simulink model "tqdtqr_rebuild_V3"  (R2021b)
settings: Solver=VariableStepAuto  StartTime=0.0  StopTime=10.0  RelTol=1e-3
undefined symbols (not defined in the file): ATQD_AfterTqMinGain_X_Deg, ATQD_APSCreepBaseTqD_X_kph, ATQD_APSCreepBaseTqD_Y_Deg, ATQD_APSCreepBaseTqR_X_kph, ATQD_APSCreepBaseTqR_Y_Deg, ATQD_APSCreepIterm_X_kph, ATQD_APSCreepIterm_Y_kph, ATQD_APSCreepPterm_X_kph, ATQD_APSCreepPterm_Y_kph, ATQD_APSDecReq_X_kph, ATQD_APSDecReq_Y_mps2, ATQD_APSDecReqCMD_X_kph, ATQD_APSDecReqTs_X_pct, ATQD_APSDecTimeGain_X_Deg, ATQD_APSDecTimeGain_Y_s, ATQD_APSReqLowSpd_X_Deg, ATQD_AutoHoldReleaseBPS_X_Deg, ATQD_AWDLoadTrqnsGain_X_kg, ATQD_AWDLoadTrqnsGain_Y_pct, ATQD_BOSEnBPSPosn_X_kph, ATQD_BOSMap_X_rpm, ATQD_BOSMap_Y_pct, ATQD_CreepBaseTqD_X_kph, ATQD_CreepBaseTqD_Y_Deg, ATQD_CreepBaseTqR_X_kph, ATQD_CreepBaseTqR_Y_Deg, ATQD_CreepBPSDisPosn_X_Deg, ATQD_CreepBPSDisPosnR_X_Deg, ATQD_CreepBPSEnPosn_X_Deg, ATQD_CreepBPSEnPosnR_X_Deg, ATQD_CreepDeltaTq_X_kph, ATQD_CreepIterm_X_kph, ATQD_CreepIterm_Y_kph, ATQD_CreepItermMaxLimit_X_pct, ATQD_CreepPreloadTime_X_kph, ATQD_CreepPreloadTq_X_kph, ATQD_CreepPreloadTq_Y_s, ATQD_CreepProtTq_X_Deg, ATQD_CreepPterm_X_kph, ATQD_CreepPterm_Y_kph, ATQD_CreepRrTqSpRat_X_rpm, ATQD_CreepRrTqSpRat_Y_Nm, ATQD_CreepTargetSpdD_X_pct, ATQD_CreepTargetSpdR_X_pct, ATQD_CreepUpLimitTq_X_rpm, ATQD_DecIneOPDHoldEnDelay_X_Deg, ATQD_DecIneOPDHoldEnDelay_Y_bar, ATQD_ECOTqMapD_X_rpm, ATQD_ECOTqMapD_Y_pct, ATQD_EMTqMapD_X_rpm, ATQD_EMTqMapD_Y_pct, ATQD_EOPDTqMapDCon_X_rpm, ATQD_EOPDTqMapDCon_Y_Deg, ATQD_EstInitVehWeight_X_c, ATQD_FAfterTqCMDGain_X_rpm, ATQD_FAfterTqCMDGain_Y_pct, ATQD_ForceLowSpd_X_Deg, ATQD_ForcePLimitSpd_X_Deg, ATQD_FrLossMAPLowV_X_rpm, ATQD_FrLossMAPLowV_Y_Nm ... (+949)
libraries: simulink x235, hcu_lib x208, tqr x63, tqd x6
(part 15 of 37)

== system tqdtqr_rebuild_V3/Input_Convert/Main function/AvaliableTqLimit function/TorqueCapacityCalcalation ==
  VTQD_FrShaftSpd_rpm : Inport
  VTQD_RrShaftSpd_rpm : Inport  Port=2
  VINP_HVBPwrAvailDchrg_kw : Inport  Port=3
  VINP_HVBPwrAvailChrg_kw : Inport  Port=4
  KTQD_FrBatapCont_factor : Inport  Port=5
  KTQD_RrBatapCont_factor : Inport  Port=6
  VTQD_FrEDUSpRat_cmd : Inport  Port=7
  VTQD_RrEDUSpRat_rat : Inport  Port=8
  VINP_FrMotorAvailTq_Nm : Inport  Port=9
  VINP_RrMotorAvailTq_Nm : Inport  Port=10
  VINP_FrRegenAvailTq_Nm : Inport  Port=11
  VINP_RrRegenAvailTq_Nm : Inport  Port=12
  VTQD_GearActualPosn_enum : Inport  Port=13
  VINP_VehicleType_enum : Inport  Port=14
  VTQD_CoordWhlTqDemFr_Nm : Inport  Port=15
  VTQD_CoordWhlTqDemRr_Nm : Inport  Port=16
  VINP_FrMCUDCBusVolt_V : Inport  Port=17
  VINP_RrMCUDCBusVolt_V : Inport  Port=18
  VPMM_DrivetrainSelect_enum : Inport  Port=19
  VINP_FrMCUTemp_C : Inport  Port=20
  VINP_FrTMTemp_C : Inport  Port=21
  VINP_RrMCUTemp_C : Inport  Port=22
  VINP_RrTMTemp_C : Inport  Port=23
  VTQD_IVIRockModeEn_flg : Inport  Port=24
  VTQD_ActAPSPosn_pct : Inport  Port=25
  task_time_s : Inport  Port=26
  CapacityDistribution : Subsystem
  Constant1 : Constant  Value=KTQD_RockInitMotTqInc_Nm
  Constant10 : Constant  Value=KTQD_RrUppTheldTrq_Nm
  Constant11 : Constant  Value=KTQD_RrUppTheldTrq_Nm
  Constant12 : Constant  Value=KTQD_RockInitTqMotDec_Nm
  Constant13 : Constant  Value=KTQD_RockAvalMotTqReset_pct
  Constant14 : Constant  Value=KTQD_RockAvalMotTqReset_pct
  Constant2 : Constant  Value=KTQD_FrRockAvalMotTqInc_Nm
  Constant3 : Constant  Value=KTQD_FrRockAvalMotBaseTq_Nm
  Constant4 : Constant  Value=KTQD_FrUppTheldTrq_Nm
  Constant5 : Constant  Value=KTQD_FrUppTheldTrq_Nm
  Constant6 : Constant  Value=KTQD_RockInitTqMotDec_Nm
  Constant7 : Constant  Value=KTQD_RockInitMotTqInc_Nm
  Constant8 : Constant  Value=KTQD_RrRockAvalMotTqInc_Nm
  Constant9 : Constant  Value=KTQD_RrRockAvalMotBaseTq_Nm
  Generation : tqd/TQD/TorqueDemand/TorqueModule/AvaliableTqLimit/TorqueCapacityCalcalation/Generation  SystemSampleTime=-1  VariantActivationTime=update diagram  Latency=0  AutoFrameSizeCalculation=off
  KTQD_FrMotorTempHigh_C KTQD_FrMotorTempLow_C : Relay  OnSwitchValue=KTQD_FrMotorTempHigh_C  OffSwitchValue=KTQD_FrMotorTempLow_C  OutDataTypeStr=boolean
  KTQD_RrMotorTempHigh_C KTQD_RrMotorTempLow_C : Relay  OnSwitchValue=KTQD_RrMotorTempHigh_C  OffSwitchValue=KTQD_RrMotorTempLow_C  OutDataTypeStr=boolean
  "MOTOR Loss MAP " : Subsystem
  MTQD_FrGenActReduce_Z_Nm : Lookup_n-D  BreakpointsForDimension1=ATQD_FrMotActReduce_Y_C  BreakpointsForDimension2=ATQD_FrMotActReduce_X_rpm  Table=MTQD_FrGenActReduce_Z_Nm  InternalRulePriority=Speed  RndMeth=Simplest  InputSameDT=on
      settings: InputPortMap=u0,u1
  MTQD_FrMotActReduce_Z_Nm : Lookup_n-D  BreakpointsForDimension1=ATQD_FrMotActReduce_Y_C  BreakpointsForDimension2=ATQD_FrMotActReduce_X_rpm  Table=MTQD_FrMotActReduce_Z_Nm  InternalRulePriority=Speed  RndMeth=Simplest  InputSameDT=on
      settings: InputPortMap=u0,u1
  MTQD_RrGenActReduce_Z_Nm : Lookup_n-D  BreakpointsForDimension1=ATQD_FrMotActReduce_Y_C  BreakpointsForDimension2=ATQD_FrMotActReduce_X_rpm  Table=MTQD_RrGenActReduce_Z_Nm  InternalRulePriority=Speed  RndMeth=Simplest  InputSameDT=on
      settings: InputPortMap=u0,u1
  MTQD_RrMotActReduce_Z_Nm : Lookup_n-D  BreakpointsForDimension1=ATQD_FrMotActReduce_Y_C  BreakpointsForDimension2=ATQD_FrMotActReduce_X_rpm  Table=MTQD_RrMotActReduce_Z_Nm  InternalRulePriority=Speed  RndMeth=Simplest  InputSameDT=on
      settings: InputPortMap=u0,u1
  Max{,1..7} (8 alike) : MinMax  Function=max  Inputs=2
  Motoring : tqd/TQD/TorqueDemand/TorqueModule/AvaliableTqLimit/TorqueCapacityCalcalation/Motoring  SystemSampleTime=-1  VariantActivationTime=update diagram  Latency=0  AutoFrameSizeCalculation=off
  OR : Logic  Operator=OR  AllPortsSameDT=off  OutDataTypeStr=boolean
  OR1 : Logic  Operator=OR  AllPortsSameDT=off  OutDataTypeStr=boolean
  RateLimit : hcu_lib/Basic_Blocks/RateLimit
  RateLimit1 : hcu_lib/Basic_Blocks/RateLimit
  Relational Operator : RelationalOperator  Operator=<=  OutDataTypeStr=boolean  RndMeth=Simplest
  Relational Operator1 : RelationalOperator  Operator=<=  OutDataTypeStr=boolean  RndMeth=Simplest
  Switch{,1..3} (4 alike) : Switch  Criteria=u2 ~= 0
      settings: AttributesFormatString=%<Criteria>
  TMAvailablePwr_Calculation : Subsystem
  VTQD_WhlTqCapMotFr_Nm : Outport
  VTQD_WhlTqCapMotRr_Nm : Outport  Port=2
  VTQD_WhlTqCapGenFr_Nm : Outport  Port=3
  VTQD_WhlTqCapGenRr_Nm : Outport  Port=4
  VTQD_MotorLossTotal_kw : Outport  Port=5
  wires:
  [VTQD_TMPwrAvailDchrg_kW] -> CapacityDistribution/3(VTQD_TMPwrAvailDchrg_kW)
  TMAvailablePwr_Calculation/1(VTQD_TMPwrAvailDchrg_kW) -> [VTQD_TMPwrAvailDchrg_kW]
  [VINP_HVBPwrAvailDchrg_kw] -> TMAvailablePwr_Calculation/1(VINP_HVBPwrAvailDchrg_kw)
  Motoring/2 -> VTQD_WhlTqCapMotRr_Nm/1
  [VTQD_RrEDUSpRat_rat] -> CapacityDistribution/2(VTQD_RrEDUSpRat_rat)
  [VTQD_FrEDUSpRat_rat] -> CapacityDistribution/1(VTQD_FrEDUSpRat_cmd)
  CapacityDistribution/4(VTQD_RrHVBPwrAvailChrg_kw) -> [VTQD_RrHVBPwrAvailChrg_kw]
  CapacityDistribution/3(VTQD_FrHVBPwrAvailChrg_kw) -> [VTQD_FrHVBPwrAvailChrg_kw]
  CapacityDistribution/2(VTQD_RrHVBPwrAvailDchrg_kw) -> [VTQD_RrHVBPwrAvailDchrg_kw]
  CapacityDistribution/1(VTQD_FrHVBPwrAvailDchrg_kw) -> [VTQD_FrHVBPwrAvailDchrg_kw]
  [VINP_HVBPwrAvailChrg_kw] -> CapacityDistribution/4(VINP_HVBPwrAvailChrg_kw)
  Generation/1 -> VTQD_WhlTqCapGenFr_Nm/1
  VTQD_RrEDUSpRat_rat/1 -> [VTQD_RrEDUSpRat_rat]
  VTQD_FrEDUSpRat_cmd/1 -> [VTQD_FrEDUSpRat_rat]
  KTQD_RrBatapCont_factor/1 -> [KTQD_RrBatapCont_factor]
  VTQD_RrShaftSpd_rpm/1 -> [VTQD_RrShaftSpd_rpm]
  VTQD_FrShaftSpd_rpm/1 -> [VTQD_FrShaftSpd_rpm]
  VINP_HVBPwrAvailChrg_kw/1 -> [VINP_HVBPwrAvailChrg_kw]
  VINP_HVBPwrAvailDchrg_kw/1 -> [VINP_HVBPwrAvailDchrg_kw]
  KTQD_FrBatapCont_factor/1 -> [KTQD_FrBatapCont_factor]
  Motoring/1 -> VTQD_WhlTqCapMotFr_Nm/1
  VINP_RrRegenAvailTq_Nm/1 -> [VINP_RrRegenAvailTq_Nm]
  VINP_FrRegenAvailTq_Nm/1 -> [VINP_FrRegenAvailTq_Nm]
  VINP_FrMotorAvailTq_Nm/1 -> [VINP_FrMotorAvailTq_Nm]
  VINP_RrMotorAvailTq_Nm/1 -> [VINP_RrMotorAvailTq_Nm]
  VTQD_GearActualPosn_enum/1 -> [VTQD_GearActualPosn_enum]
  VINP_VehicleType_enum/1 -> [VINP_VehicleType_enum]
  [VTQD_FrShaftSpd_rpm] -> "MOTOR Loss MAP "/1(VTQD_FrShaftSpd_rpm)
  [VTQD_RrShaftSpd_rpm] -> "MOTOR Loss MAP "/2(VTQD_RrShaftSpd_rpm)
  [VTQD_CoordWhlTqDemFr_Nm] -> "MOTOR Loss MAP "/3(VTQD_CoordWhlTqDemFr_Nm)
  [VTQD_CoordWhlTqDemRr_Nm] -> "MOTOR Loss MAP "/4(VTQD_CoordWhlTqDemRr_Nm)
  [VINP_FrMCUDCBusVolt_V] -> "MOTOR Loss MAP "/5(VINP_FrMCUDCBusVolt_V)
  [VINP_RrMCUDCBusVolt_V] -> "MOTOR Loss MAP "/6(VINP_RrMCUDCBusVolt_V)
  [VPMM_DrivetrainSelect_enum] -> "MOTOR Loss MAP "/7(VPMM_DrivetrainSelect_enum)
  VTQD_CoordWhlTqDemRr_Nm/1 -> [VTQD_CoordWhlTqDemRr_Nm]
  VTQD_CoordWhlTqDemFr_Nm/1 -> [VTQD_CoordWhlTqDemFr_Nm]
  VINP_FrMCUDCBusVolt_V/1 -> [VINP_FrMCUDCBusVolt_V]
  VINP_RrMCUDCBusVolt_V/1 -> [VINP_RrMCUDCBusVolt_V]
  VPMM_DrivetrainSelect_enum/1 -> [VPMM_DrivetrainSelect_enum]
  "MOTOR Loss MAP "/1(VTQD_MotorLossTotal_kW) -> VTQD_MotorLossTotal_kw/1, [VTQD_MotorLossTotal_kw]
  [VTQD_MotorLossTotal_kw] -> CapacityDistribution/5(VTQD_MotorLossTotal_kw)
  VINP_FrMCUTemp_C/1 -> [VINP_FrMCUTemp_C]
  VINP_FrTMTemp_C/1 -> [VINP_FrTMTemp_C]
  VINP_RrMCUTemp_C/1 -> [VINP_RrMCUTemp_C]
  VINP_RrTMTemp_C/1 -> [VINP_RrTMTemp_C]
  [VTQD_CoordWhlTqDemFr_Nm] -> Max6/2
  Constant3/1 -> Max6/1
  Max6/1 -> Switch/1
  [VTQD_IVIRockModeEn_flg] -> Switch/2
  OR/1 -> Switch1/2
  [VTQD_IVIRockModeEn_flg] -> OR/1
  Constant1/1 -> Switch1/1
  Constant2/1 -> Switch1/3
  Switch/1 -> [VTQD_FrRockDisAvalMotInpTq_Nm]  "VTQD_FrRockDisAvalMotInpTq_Nm"
  Switch1/1 -> [VTQD_FrRockAvalMotTqInc_Nm]  "VTQD_FrRockAvalMotTqInc_Nm"
  [VTQD_FrRockDisAvalMotInpTq_Nm] -> RateLimit/1
  Constant4/1 -> Switch/3
  Constant5/1 -> RateLimit/2
  [task_time_s] -> RateLimit/3
  [VTQD_FrRockAvalMotTqInc_Nm] -> RateLimit/4
  Constant6/1 -> RateLimit/5
  RateLimit/1 -> [VTQD_FrRockDisAvalMotTq_Nm]  "VTQD_FrRockDisAvalMotTq_Nm"
  RateLimit1/1 -> [VTQD_RrRockDisAvalMotTq_Nm]  "VTQD_RrRockDisAvalMotTq_Nm"
  Constant12/1 -> RateLimit1/5
  [VTQD_RrRockAvalMotTqInc_Nm] -> RateLimit1/4
  [task_time_s] -> RateLimit1/3
  Constant11/1 -> RateLimit1/2
  Constant10/1 -> Switch2/3
  [VTQD_RrRockDisAvalMotInpTq_Nm] -> RateLimit1/1
  Switch3/1 -> [VTQD_RrRockAvalMotTqInc_Nm]  "VTQD_RrRockAvalMotTqInc_Nm"
  Switch2/1 -> [VTQD_RrRockDisAvalMotInpTq_Nm]  "VTQD_RrRockDisAvalMotInpTq_Nm"
  Constant8/1 -> Switch3/3
  Constant7/1 -> Switch3/1
  [VTQD_IVIRockModeEn_flg] -> Switch2/2
  Max7/1 -> Switch2/1
  Constant9/1 -> Max7/1
  [VTQD_CoordWhlTqDemRr_Nm] -> Max7/2
  Relational Operator/1 -> OR/2
  [VTQD_ActAPSPosn_pct] -> Relational Operator/1
  Constant13/1 -> Relational Operator/2
  [VTQD_ActAPSPosn_pct] -> Relational Operator1/1
  OR1/1 -> Switch3/2
  [VTQD_IVIRockModeEn_flg] -> OR1/1
  Constant14/1 -> Relational Operator1/2
  Relational Operator1/1 -> OR1/2
  MTQD_FrMotActReduce_Z_Nm/1 -> [VTQD_FrMotActReduce_Nm]  "VTQD_FrMotActReduce_Nm"
  [VINP_FrTMTemp_C] -> Max/2
  KTQD_FrMotorTempHigh_C KTQD_FrMotorTempLow_C/1 -> [VTQD_FrMotorTempHigh_flg]  "VTQD_FrMotorTempHigh_flg"
  Max/1 -> KTQD_FrMotorTempHigh_C KTQD_FrMotorTempLow_C/1
  Max1/1 -> KTQD_RrMotorTempHigh_C KTQD_RrMotorTempLow_C/1
  [VTQD_RrShaftSpd_rpm] -> MTQD_RrGenActReduce_Z_Nm/2
  Max4/1 -> MTQD_RrMotActReduce_Z_Nm/1
  MTQD_RrMotActReduce_Z_Nm/1 -> [VTQD_RrMotActReduce_Nm]  "VTQD_RrMotActReduce_Nm"
  [VINP_FrTMTemp_C] -> Max3/2
  KTQD_RrMotorTempHigh_C KTQD_RrMotorTempLow_C/1 -> [VTQD_RrMotorTempHigh_flg]  "VTQD_RrMotorTempHigh_flg"
  MTQD_RrGenActReduce_Z_Nm/1 -> [VTQD_RrGenActReduce_Nm]  "VTQD_RrGenActReduce_Nm"
  Max2/1 -> MTQD_FrMotActReduce_Z_Nm/1
  MTQD_FrGenActReduce_Z_Nm/1 -> [VTQD_FrGenActReduce_Nm]  "VTQD_FrGenActReduce_Nm"
  [VINP_RrMCUTemp_C] -> Max1/1
  [VTQD_FrShaftSpd_rpm] -> MTQD_FrGenActReduce_Z_Nm/2
  [VINP_RrTMTemp_C] -> Max1/2
  [VINP_RrMCUTemp_C] -> Max5/1
  [VINP_RrTMTemp_C] -> Max5/2
  [VINP_FrMCUTemp_C] -> Max3/1
  Max3/1 -> MTQD_FrGenActReduce_Z_Nm/1
  [VINP_FrTMTemp_C] -> Max2/2
  [VTQD_FrShaftSpd_rpm] -> MTQD_FrMotActReduce_Z_Nm/2
  [VINP_FrMCUTemp_C] -> Max2/1
  [VTQD_RrShaftSpd_rpm] -> MTQD_RrMotActReduce_Z_Nm/2
  [VINP_RrTMTemp_C] -> Max4/2
  Max5/1 -> MTQD_RrGenActReduce_Z_Nm/1
  [VINP_RrMCUTemp_C] -> Max4/1
  [VINP_FrMCUTemp_C] -> Max/1
  [VTQD_FrRockDisAvalMotTq_Nm] -> Motoring/15
  [VTQD_RrRockDisAvalMotTq_Nm] -> Motoring/16
  [VTQD_FrMotActReduce_Nm] -> Motoring/13
  [VTQD_RrMotorTempHigh_flg] -> Motoring/12
  [VINP_FrMotorAvailTq_Nm] -> Motoring/7
  [VTQD_RrMotActReduce_Nm] -> Motoring/14
  [VTQD_FrMotorTempHigh_flg] -> Motoring/11
  [VINP_VehicleType_enum] -> Motoring/10
  [VTQD_GearActualPosn_enum] -> Motoring/9
  [VINP_RrMotorAvailTq_Nm] -> Motoring/8
  [KTQD_FrBatapCont_factor] -> Motoring/5
  [KTQD_RrBatapCont_factor] -> Motoring/6
  [VTQD_RrHVBPwrAvailDchrg_kw] -> Motoring/4
  [VTQD_RrShaftSpd_rpm] -> Motoring/2
  [VTQD_FrHVBPwrAvailDchrg_kw] -> Motoring/3
  [VTQD_FrShaftSpd_rpm] -> Motoring/1
  VTQD_IVIRockModeEn_flg/1 -> [VTQD_IVIRockModeEn_flg]
  VTQD_ActAPSPosn_pct/1 -> [VTQD_ActAPSPosn_pct]
  task_time_s/1 -> [task_time_s]
  [VTQD_RrShaftSpd_rpm] -> Generation/2
  [VTQD_FrGenActReduce_Nm] -> Generation/13
  [VTQD_FrMotorTempHigh_flg] -> Generation/11
  [VTQD_RrMotorTempHigh_flg] -> Generation/12
  [VTQD_GearActualPosn_enum] -> Generation/9
  [VINP_VehicleType_enum] -> Generation/10
  [VINP_RrRegenAvailTq_Nm] -> Generation/8
  [VTQD_FrHVBPwrAvailChrg_kw] -> Generation/3
  [KTQD_FrBatapCont_factor] -> Generation/5
  [KTQD_RrBatapCont_factor] -> Generation/6
  [VTQD_FrShaftSpd_rpm] -> Generation/1
  [VTQD_RrHVBPwrAvailChrg_kw] -> Generation/4
  [VINP_FrRegenAvailTq_Nm] -> Generation/7
  [VTQD_RrGenActReduce_Nm] -> Generation/14
  Generation/2 -> VTQD_WhlTqCapGenRr_Nm/1

== system tqdtqr_rebuild_V3/Input_Convert/Main function/DriverWhlTqDem function/BOS ==
  note: Calculate BOS torque
  note: BOS enable conditions
  BSCPIn_outputs : Inport
  BSignalConvert_outputs : Inport  Port=2
  BFunction_outputs : Inport  Port=3
  VTQD_PedalMapWhlTq_Nm : Inport  Port=4
  VTQD_CreepBaseTqR_Nm : Inport  Port=5
  VTQD_CreepBaseTqD_Nm : Inport  Port=6
  VTQD_HighBPSPosn_flg : Inport  Port=7
  AND : Logic  Inputs=4  AllPortsSameDT=off  OutDataTypeStr=boolean
  AND1 : Logic  AllPortsSameDT=off  OutDataTypeStr=boolean
  AND2 : Logic  AllPortsSameDT=off  OutDataTypeStr=boolean
  Bus Selector : BusSelector  OutputSignals=VTQD_ActBPSPosn_pct,VVMC_APSActive_flg,VTQD_LowIdleAccPedal_flg,VTQD_LimpHomeAct_flg
  Bus Selector1 : BusSelector  OutputSignals=VTQD_TqTargetShaftSpd_rpm,VTQD_BrkSwSta_flg,VTQD_VehActSpd_kph
  Bus Selector2 : BusSelector  OutputSignals=VTQD_GearActualPosn_enum
  Constant1 : Constant  Value=KTQD_BOSEnPedalTq_Nm
  Constant18 : Constant  Value=ZERO_FLOAT
  Constant20 : Constant  Value=ENUM_GEARACTUALPOSN_R
  Constant3 : Constant  Value=ONE_PERCENT
  Constant96 : Constant  Value=KTQD_FailsafeActiveSW_flg
  Detect Change : simulink/Logic and Bit Operations/Detect Change  vinit=0  OutDataTypeStr=boolean
  Equal10 : RelationalOperator  Operator===  OutDataTypeStr=boolean  RndMeth=Simplest
  Logical Operator13 : Logic  AllPortsSameDT=off  OutDataTypeStr=boolean
  MTQD_BOSEnBPSPosn_Y_pct : Lookup_n-D  NumberOfTableDimensions=1  BreakpointsForDimension1=ATQD_BOSEnBPSPosn_X_kph  Table=MTQD_BOSEnBPSPosn_Y_pct  InternalRulePriority=Speed  RndMeth=Simplest  InputSameDT=on
  MTQD_BOSMap_Z_pct : Lookup_n-D  BreakpointsForDimension1=ATQD_BOSMap_Y_pct  BreakpointsForDimension2=ATQD_BOSMap_X_rpm  Table=MTQD_BOSMap_Z_pct  ExtrapMethod=Clip  InternalRulePriority=Speed  RndMeth=Simplest  InputSameDT=on
      settings: InputPortMap=u0,u1
  Max : MinMax  Function=max  Inputs=2
  NOT{,1..3} (4 alike) : Logic  Operator=NOT  AllPortsSameDT=off  OutDataTypeStr=boolean
  OR : Logic  Operator=OR  Inputs=3  AllPortsSameDT=off  OutDataTypeStr=boolean
  OR1 : Logic  Operator=OR  AllPortsSameDT=off  OutDataTypeStr=boolean
  OR2 : Logic  Operator=OR  AllPortsSameDT=off  OutDataTypeStr=boolean
  Product1 : Product  RndMeth=Zero
  Product2 : Product  RndMeth=Zero
  Product3 : Product  RndMeth=Zero
  Relational Operator : RelationalOperator  Operator=>  OutDataTypeStr=boolean  RndMeth=Simplest
  Relational Operator1 : RelationalOperator  Operator=>  OutDataTypeStr=boolean  RndMeth=Simplest
  Relational Operator2 : RelationalOperator  OutDataTypeStr=boolean  RndMeth=Simplest
  Relational Operator5 : RelationalOperator  Operator=>  OutDataTypeStr=boolean  RndMeth=Simplest
  SR_Latch : hcu_lib/Basic_Blocks/SR_Latch
  Switch7 : Switch  Criteria=u2 ~= 0
      settings: AttributesFormatString=%<Criteria>
  Switch8 : Switch  Criteria=u2 ~= 0
      settings: AttributesFormatString=%<Criteria>
  VTQD_BOSEnable_flg : Outport
  VTQD_BOSTq_Nm : Outport  Port=2
  wires:
  [VTQD_ActBPSPosn_pct] -> MTQD_BOSMap_Z_pct/1
  [VTQD_TqTargetShaftSpd_rpm] -> MTQD_BOSMap_Z_pct/2
  Constant3/1 -> Product1/2
  Product1/1 -> [VTQD_BOSReduction_gain]  "VTQD_BOSReduction_gain"
  MTQD_BOSMap_Z_pct/1 -> Product1/1
  Relational Operator/1 -> AND/1
  [VTQD_VehActSpd_kph] -> MTQD_BOSEnBPSPosn_Y_pct/1
  MTQD_BOSEnBPSPosn_Y_pct/1 -> Relational Operator/2  "VTQD_BOSEnBPSPosn_pct"
  [VTQD_ActBPSPosn_pct] -> Relational Operator/1
  VTQD_PedalMapWhlTq_Nm/1 -> [VTQD_PedalMapWhlTq_Nm]
  Relational Operator1/1 -> AND/2
  [VTQD_PedalMapWhlTq_Nm] -> Relational Operator1/1
  Constant1/1 -> Relational Operator1/2
  [VTQD_PedalMapWhlTq_Nm] -> Product2/1
  [VTQD_BOSReduction_gain] -> Product2/2
  Product3/1 -> Max/2
  Switch8/1 -> VTQD_BOSTq_Nm/1, [VTQD_BOSTq_Nm]  "VTQD_BOSTq_Nm"
  [VTQD_CreepBaseTqR_Nm] -> Switch7/1
  Max/1 -> Switch8/1
  Product2/1 -> Switch8/3
  Equal10/1 -> Switch7/2
  [VTQD_PedalMapWhlTq_Nm] -> Product3/1
  [VTQD_BOSReduction_gain] -> Product3/2
  [VTQD_GearActualPosn_enum] -> Equal10/1
  Relational Operator5/1 -> Switch8/2
  Constant20/1 -> Equal10/2
  Switch7/1 -> Max/1
  Constant18/1 -> Relational Operator5/2
  [VTQD_CreepBaseTqD_Nm] -> Switch7/3
  VTQD_CreepBaseTqD_Nm/1 -> [VTQD_CreepBaseTqD_Nm]
  VTQD_CreepBaseTqR_Nm/1 -> [VTQD_CreepBaseTqR_Nm]
  [VTQD_BOSReduction_gain] -> Relational Operator5/1
  NOT/1 -> AND/3
  [VVMC_APSActive_flg] -> NOT/1
  [VTQD_LowIdleAccPedal_flg] -> NOT2/1
  NOT2/1 -> AND/4
  [VTQD_BrkSwSta_flg] -> NOT3/1
  AND2/1 -> OR/3
  AND1/1 -> OR1/1
  Detect Change/1 -> OR1/2
  Relational Operator2/1 -> OR/1
  [VTQD_LowIdleAccPedal_flg] -> AND2/1
  [VTQD_GearActualPosn_enum] -> Detect Change/1
  NOT3/1 -> AND2/2
  SR_Latch/1 -> VTQD_BOSEnable_flg/1  "VTQD_BOSEnable_flg"
  AND/1 -> NOT1/1, SR_Latch/1
  [VTQD_HighBPSPosn_flg] -> OR/2
  OR/1 -> AND1/2
  NOT1/1 -> AND1/1
  [VTQD_PedalMapWhlTq_Nm] -> Relational Operator2/1
  [VTQD_BOSTq_Nm] -> Relational Operator2/2
  VTQD_HighBPSPosn_flg/1 -> [VTQD_HighBPSPosn_flg]
  Logical Operator13/1 -> OR2/2
  Constant96/1 -> Logical Operator13/2
  [VTQD_LimpHomeAct_flg] -> Logical Operator13/1
  OR1/1 -> OR2/1
  OR2/1 -> SR_Latch/2
  BSCPIn_outputs/1 -> Bus Selector/1
  BSignalConvert_outputs/1 -> Bus Selector1/1
  BFunction_outputs/1 -> Bus Selector2/1
  Bus Selector/1 -> [VTQD_ActBPSPosn_pct]  "<VTQD_ActBPSPosn_pct>"
  Bus Selector1/1 -> [VTQD_TqTargetShaftSpd_rpm]  "<VTQD_TqTargetShaftSpd_rpm>"
  Bus Selector2/1 -> [VTQD_GearActualPosn_enum]  "<VTQD_GearActualPosn_enum>"
  Bus Selector/2 -> [VVMC_APSActive_flg]  "<VVMC_APSActive_flg>"
  Bus Selector/3 -> [VTQD_LowIdleAccPedal_flg]  "<VTQD_LowIdleAccPedal_flg>"
  Bus Selector1/2 -> [VTQD_BrkSwSta_flg]  "<VTQD_BrkSwSta_flg>"
  Bus Selector/4 -> [VTQD_LimpHomeAct_flg]  "<VTQD_LimpHomeAct_flg>"
  Bus Selector1/3 -> [VTQD_VehActSpd_kph]  "<VTQD_VehActSpd_kph>"
